simulink model "DC_motor"  (R2016a)
settings: Solver=VariableStepAuto  StartTime=0.0  StopTime=10.0  RelTol=1e-3
values from neighbouring files (symbols this model uses):
  den = [La*J  (La*B + Ra*J)  (Ra*B+Kb*K)]    [ini.m]
  Kd = 2.6527    [ini.m]
  Ki = 26.0414    [ini.m]
  Kp = 16.6228    [ini.m]
  num = K    (= 0.015)    [ini.m]
settings Model: Creator=EBUKA  LastModifiedBy=EBUKA
settings GRTTargetCC: GeneratePreprocessorConditionals=Use local settings

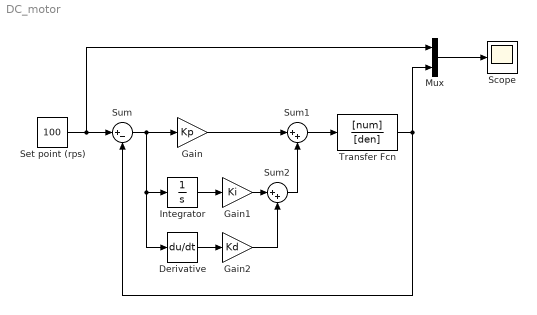
== system DC_motor ==
  Derivative : Derivative
  Gain : Gain  Gain=Kp
  Gain1 : Gain  Gain=Ki
  Gain2 : Gain  Gain=Kd
  Integrator : Integrator
  Mux : Mux  Inputs=2
  Scope : Scope
  Set point (rps) : Constant  Value=100
  Sum : Sum  Inputs=|+-
  Sum1 : Sum  Inputs=|++
  Sum2 : Sum  Inputs=|++
  Transfer Fcn : TransferFcn  Numerator=[num]  Denominator=[den]
  wires:
  Set point (rps)/1 -> Mux/1, Sum/1
  Transfer Fcn/1 -> Mux/2, Sum/2
  Mux/1 -> Scope/1
  Sum/1 -> Derivative/1, Integrator/1, Gain/1
  Sum1/1 -> Transfer Fcn/1
  Gain/1 -> Sum1/1
  Integrator/1 -> Gain1/1
  Gain1/1 -> Sum2/1
  Sum2/1 -> Sum1/2
  Derivative/1 -> Gain2/1
  Gain2/1 -> Sum2/2
